simulink model "cascade_filter"  (R2020b)
settings: Solver=FixedStepAuto  StartTime=0.0  StopTime=10.0  FixedStep=0.2  RelTol=1e-3
settings Model: Creator=Abhinav dixit  LastModifiedBy=Abhinav dixit
settings DataIOCC: SaveOutput=off  SaveTime=off

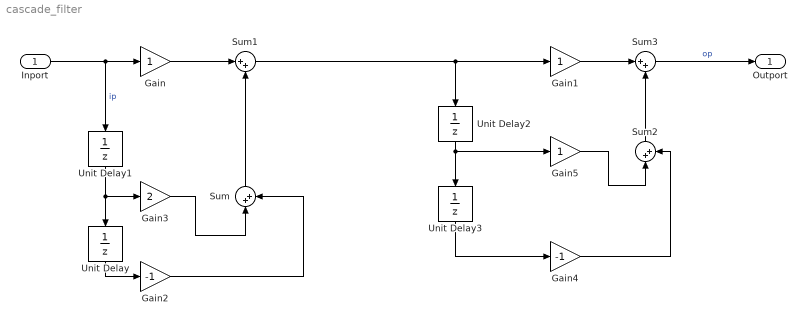
== system cascade_filter ==
  Inport : Inport  OutDataTypeStr=double  PortDimensions=1  SampleTime=[0.20000000000000001,0]
  Gain : Gain
  Gain1 : Gain
  Gain2 : Gain  Gain=-1
  Gain3 : Gain  Gain=2
  Gain4 : Gain  Gain=-1
  Gain5 : Gain
  Sum{,1..3} (4 alike) : Sum  Inputs=|++
  Unit Delay{,1..3} (4 alike) : UnitDelay  SampleTime=-1  HasFrameUpgradeWarning=on
  Outport : Outport  OutDataTypeStr=double  PortDimensions=1  SampleTime=[0.20000000000000001,0]
  wires:
  Sum1/1 -> Gain1/1, Unit Delay2/1
  Unit Delay3/1 -> Gain4/1
  Unit Delay2/1 -> Gain5/1, Unit Delay3/1
  Gain5/1 -> Sum2/1
  Sum2/1 -> Sum3/2
  Gain/1 -> Sum1/1
  Unit Delay1/1 -> Unit Delay/1, Gain3/1
  Sum3/1 -> Outport/1  "op"
  Unit Delay/1 -> Gain2/1
  Sum/1 -> Sum1/2
  Inport/1 -> Gain/1, Unit Delay1/1  "ip"
  Gain2/1 -> Sum/2
  Gain4/1 -> Sum2/2
  Gain3/1 -> Sum/1
  Gain1/1 -> Sum3/1
